simulink model "DiscreteBaseControl"  (R2022a)
settings: Solver=VariableStepAuto  StartTime=0.0  StopTime=30  RelTol=1e-3
values from neighbouring files (symbols this model uses):
  den = [1 2 1]    [DiscreteProcess.m]    (also in RTS.m = ro*poly2sym(Az, z)*poly2sym(flip(Az), z))
  input_noise_amplitude = 0    [DiscreteProcess.m]
  input_noise_time = 0    [DiscreteProcess.m]
  num = 2    [DiscreteProcess.m]    (also in RTS.m = num + den)
  PROPORTIONAL_GAIN = controller_parameters.Kp    [DiscreteProcess.m]
  reference_amplitude = 0    [DiscreteProcess.m]
  sample_time = 0.1    [DiscreteProcess.m]
undefined symbols (not defined in the file or in its folder): DiscIntNeverNeededParam
libraries: simulink x1
settings Model: Creator=natha  LastModifiedBy=lucas
settings DataIOCC: ReturnWorkspaceOutputs=off

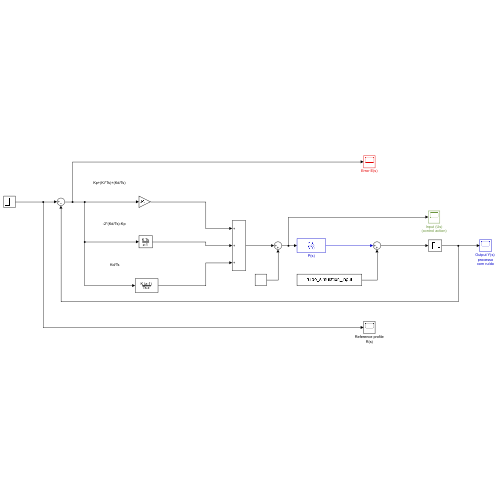
[thumbnail: Simulink's stored preview of the top-level diagram]
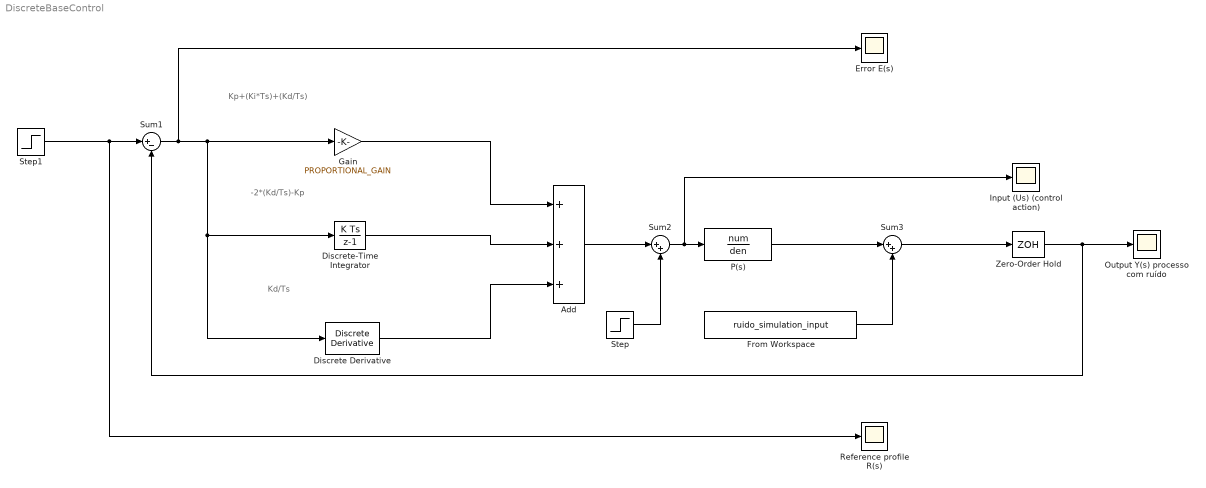
== system DiscreteBaseControl ==
  note: Kd/Ts
  note: -2*(Kd/Ts)-Kp
  note: Kp+(Ki*Ts)+(Kd/Ts)
  Add : Sum  Inputs=+++
  Discrete Derivative : simulink/Discrete/Discrete Derivative  gainval=DERIVATIVE_GAIN  ICPrevScaledInput=0.0  OutMin=[]  OutMax=[]  OutDataType=fixdt(1, 16)  OutScaling=2^-10  DoSatur=off
  Discrete-Time Integrator : DiscreteIntegrator  gainval=INTEGRAL_GAIN  SampleTime=sample_time  ICPrevOutput=DiscIntNeverNeededParam  ICPrevScaledInput=DiscIntNeverNeededParam
  Error E(s) : Scope
  From Workspace : FromWorkspace  VariableName=ruido_simulation_input  SampleTime=sample_time
  Gain : Gain  Gain=PROPORTIONAL_GAIN
  Input (Us) (control action) : Scope
  Output Y(s) processo com ruído : Scope
  P(s) : TransferFcn  Numerator=num  Denominator=den
  Reference profile R(s) : Scope
  Step : Step  Time=input_noise_time  After=input_noise_amplitude  SampleTime=sample_time
  Step1 : Step  Time=0  After=reference_amplitude  SampleTime=0
  Sum1 : Sum  Inputs=|+-
  Sum2 : Sum  Inputs=|++
  Sum3 : Sum  Inputs=|++
  Zero-Order Hold : ZeroOrderHold  SampleTime=sample_time
  wires:
  Step1/1 -> Reference profile R(s)/1, Sum1/1
  Sum1/1 -> Error E(s)/1, Discrete Derivative/1, Discrete-Time Integrator/1, Gain/1
  Gain/1 -> Add/1
  Discrete-Time Integrator/1 -> Add/2
  Discrete Derivative/1 -> Add/3
  Add/1 -> Sum2/1
  Step/1 -> Sum2/2
  Sum2/1 -> Input (Us) (control action)/1, P(s)/1
  From Workspace/1 -> Sum3/2
  Sum3/1 -> Zero-Order Hold/1
  Zero-Order Hold/1 -> Sum1/2, Output Y(s) processo com ruído/1
  P(s)/1 -> Sum3/1
